simulink library "M160_lib"  (Simulink 7.8)
settings: Solver=FixedStepDiscrete  StartTime=0.0  StopTime=10.0  RelTol=1e-3
PreLoadFcn:
  | update_path
undefined symbols (not defined in the file): Afr_atCool2facLambdaReqCorr_CUR_x, Afr_atCool2facLambdaReqCorr_CUR_y, Afr_atMani2facLambdaReqCorr_CUR_x, Afr_atMani2facLambdaReqCorr_CUR_y, Afr_facLambdaReqMan, Afr_facRatioMan, Afr_facStoich, Afr_flgLambdaReqOverride, Afr_flgRatioOverride, Afr_rpmEngSpdfacRelAir2facLambdaReqBase_MAP_x, Afr_rpmEngSpdfacRelAir2facLambdaReqBase_MAP_y, Afr_rpmEngSpdfacRelAir2facLambdaReqBase_MAP_z, Ais_flgAirInjReacPumpOverride, Ais_stAirInjReacPumpMan, Amc_flgAirMassFlowOverride, Amc_uSens2AirMassFlow_CUR_x, Amc_uSens2AirMassFlow_CUR_y, Amc_uSensMaxValid, Amc_uSensMinValid, Amf_facRelAirMan, Amf_flgAirMassPerStrOverride, Amf_flgRelAirOverride, Amf_flgSwitch2AirMassFlowMeter, Amf_mAirPerStrMan, Amf_pManiEngSpd2facRelAirCorr_MAP_x, Amf_pManiEngSpd2facRelAirCorr_MAP_y, Amf_pManiEngSpd2facRelAirCorr_MAP_z, Amf_rpmEngSpd2facTempCorr_CUR_x, Amf_rpmEngSpd2facTempCorr_CUR_y, Amf_shcSpecGasConst_C, Amf_volEngDisp_C, Apv_facAirPumpRateMan, Apv_factor, Apv_flgAirPumpRateOverride, Apv_tiPeriod_C, Bvc_rVoltDivHigh, Bvc_rVoltDivLow, Bvc_uBattMax, Bvc_uBattMin, CDRV_E_OK_, Cov_facChOverVlvRateMan, Cov_factor, Cov_flgChOverVlvRateOverride, Cov_tiPeriod_C, Cpc_atManiTmp2facPresCorr_CUR_x, Cpc_atManiTmp2facPresCorr_CUR_y, Cpc_flgPChargeOverride, Cpc_uSens2pManiBase_CUR_x, Cpc_uSens2pManiBase_CUR_y, Ctc_rPullUp_C, Ctc_rSens2atCool_CUR_x, Ctc_rSens2atCool_CUR_y, Ctc_uSensMaxValid, Ctc_uSensMinValid, Ctc_uSupply, Doh_OutputDiagnosisOverride, dummy_facAirPumpRateReq, dummy_facChOverVlvRateReq, dummy_flgInterCoolerOverride, dummy_flgKl50Override ... (+243)
libraries: simulink x36, ehooks_lib x3
(part 4 of 8)

== system M160_lib/Sensors/Ctc ==
  function : TriggerPort  TriggerType=function-call
  Constant : Constant  Value=Ctc_rPullUp_C
  Constant3 : Constant  Value=Ctc_uSupply
  Constant6 : Constant  Value=0  OutDataTypeStr=single
  Ctc_rSens2atCool_CUR : Lookup_n-D  NumberOfTableDimensions=1  BreakpointsForDimension1=Ctc_rSens2atCool_CUR_x  BreakpointsForDimension1DataTypeStr=Inherit: Inherit from 'Breakpoint data'  Table=Ctc_rSens2atCool_CUR_y  TableDataTypeStr=Inherit: Inherit from 'Table data'  ExtrapMethod=Clip  OutDataTypeStr=Inherit: Inherit from 'Table data'  InputSameDT=on
  Divide : Product  Inputs=*/  OutDataTypeStr=Inherit: Same as first input
  G1_ADC_Input_Receive : Subsystem  LoadFcn=ehooks_medc17flex_devlib_io_block('load');  InitFcn=ehooks_medc17flex_devlib_io_block('init');  StartFcn=ehooks_medc17flex_devlib_io_block('start');  StopFcn=ehooks_medc17flex_devlib_io_block('stop');  ClipboardFcn=ehooks_medc17flex_devlib_io_block('clipboard', 0); % Second argument just needed to indicate null block. See callback handler.  mask{ChannelName=I_A_AN10}
      mask prompts: ChannelName "Channel name"
      mask init:
      | ehooks_medc17flex_devlib_io_block('mask_init');
      settings: AttributesFormatString=Channel name: '%<ChannelName>'  CopyFcn=ehooks_medc17flex_devlib_io_block('copy');  DeleteFcn=ehooks_medc17flex_devlib_io_block('delete');  UndoDeleteFcn=ehooks_medc17flex_devlib_io_block('undo_delete');  ModelCloseFcn=ehooks_medc17flex_devlib_io_block('model_close');  PreSaveFcn=ehooks_medc17flex_devlib_io_block('pre_save');  PostSaveFcn=ehooks_medc17flex_devlib_io_block('post_save');  NameChangeFcn=ehooks_medc17flex_devlib_io_block('name_change');  DestroyFcn=ehooks_medc17flex_devlib_io_block('destroy', 0); % Second argument just needed to indicate null block. See callback handler.  OpenFcn=ehooks_medc17flex_devlib_io_block('open');  CloseFcn=ehooks_medc17flex_devlib_io_block('close');  ParentCloseFcn=ehooks_medc17flex_devlib_io_block('parent_close');  MoveFcn=ehooks_medc17flex_devlib_io_block('move');
      mask StyleString: popup(<empty>|I_A_AN01|I_A_AN02|I_A_AN03|I_A_AN05|I_A_AN06|I_A_AN07|I_A_AN08|I_A_AN10|I_A_AN11|I_A_AN12|I_A_AN13|I_A_AN14|I_A_AN15|I_A_AN16|I_A_AN17|I_A_AN18|I_A_AN19|I_A_AN20|I_A_AN21|I_A_AN23|I_A_AN32|I_A_AN35|I_A_AN36|I_A_AN37|I_A_AN39|I_A_AN100|I_A_AN101|I_A_AN103|I_A_AN104|I_A_AN105|I_A_AN106)
      mask Display: image(imread('Input_Analog.jpg'))
  Interval Test : simulink/Logic and Bit Operations/Interval Test  IntervalClosedRight=on  uplimit=Ctc_uSensMaxValid  IntervalClosedLeft=on  lowlimit=Ctc_uSensMinValid  OutDataTypeStr=boolean
  Logical Operator : Logic  Operator=NOT  AllPortsSameDT=off  OutDataTypeStr=boolean
  Logical Operator1 : Logic  Operator=NOT  AllPortsSameDT=off  OutDataTypeStr=boolean
  Logical Operator2 : Logic  Operator=NOT  AllPortsSameDT=off  OutDataTypeStr=boolean
  Logical Operator4 : Logic  Operator=OR  Inputs=3  AllPortsSameDT=off  OutDataTypeStr=boolean
  Product : Product  OutDataTypeStr=Inherit: Same as first input
  Relational Operator : RelationalOperator  Operator=>  OutDataTypeStr=boolean
  Subtract : Sum  Inputs=+-  OutDataTypeStr=Inherit: Same as first input
  Switch : Switch  Threshold=1
  Unit Delay : UnitDelay  SampleTime=-1
  Ctc_flgError : Outport
  Ctc_atCool : Outport  Port=2
  wires:
  Logical Operator4/1 -> Ctc_flgError/1  "Ctc_flgError"
  Logical Operator1/1 -> Logical Operator4/2
  Logical Operator/1 -> Logical Operator4/1
  Interval Test/1 -> Logical Operator1/1
  G1_ADC_Input_Receive/2(uRaw) -> Subtract/2, Product/1, Interval Test/1  "Ctc_uSens"
  G1_ADC_Input_Receive/1(status) -> Logical Operator/1  "Ctc_stIA"
  Constant/1 -> Product/2
  Constant3/1 -> Subtract/1
  Product/1 -> Divide/1
  Subtract/1 -> Divide/2, Relational Operator/1
  Constant6/1 -> Relational Operator/2
  Relational Operator/1 -> Logical Operator2/1, Switch/2
  Logical Operator2/1 -> Logical Operator4/3
  Switch/1 -> Ctc_atCool/1, Unit Delay/1  "Ctc_atCool"
  Unit Delay/1 -> Switch/3
  Ctc_rSens2atCool_CUR/1 -> Switch/1
  Divide/1 -> Ctc_rSens2atCool_CUR/1  "Ctc_rSens"

== system M160_lib/Sensors/Egc ==
  function : TriggerPort  TriggerType=function-call
  Abs : Abs
  Add : Sum  OutDataTypeStr=Inherit: Same as first input
  Constan1 : Constant  Value=0.05  OutDataTypeStr=single
  Constan2 : Constant  Value=0.01  OutMin=0  OutDataTypeStr=single
  Constan3 : Constant  Value=0  OutDataTypeStr=single
  Constant : Constant  Value=2  OutDataTypeStr=single
  Constant1 : Constant  Value=Egc_flgEgasOverride
  Constant2 : Constant  Value=Egc_facEgasMan
  Constant3 : Constant  Value=Egc_tiTEgasFilt
  Constant4 : Constant  Value=Egc_stEgasFilt
  Divide : Product  Inputs=*/  OutDataTypeStr=Inherit: Same as first input
  Egc_uSens2facEgas1_CUR : Lookup_n-D  NumberOfTableDimensions=1  BreakpointsForDimension1=Egc_uSens2facEgas1_CUR_x  BreakpointsForDimension1DataTypeStr=Inherit: Inherit from 'Breakpoint data'  Table=Egc_uSens2facEgas1_CUR_y  TableDataTypeStr=Inherit: Inherit from 'Table data'  ExtrapMethod=Clip  OutDataTypeStr=Inherit: Inherit from 'Table data'  InputSameDT=on
  Egc_uSens2facEgas2_CUR : Lookup_n-D  NumberOfTableDimensions=1  BreakpointsForDimension1=Egc_uSens2facEgas2_CUR_x  BreakpointsForDimension1DataTypeStr=Inherit: Inherit from 'Breakpoint data'  Table=Egc_uSens2facEgas2_CUR_y  TableDataTypeStr=Inherit: Inherit from 'Table data'  ExtrapMethod=Clip  OutDataTypeStr=Inherit: Inherit from 'Table data'  InputSameDT=on
  G1_ADC_Input_Receive : Subsystem  LoadFcn=ehooks_medc17flex_devlib_io_block('load');  InitFcn=ehooks_medc17flex_devlib_io_block('init');  StartFcn=ehooks_medc17flex_devlib_io_block('start');  StopFcn=ehooks_medc17flex_devlib_io_block('stop');  ClipboardFcn=ehooks_medc17flex_devlib_io_block('clipboard', 0); % Second argument just needed to indicate null block. See callback handler.  mask{ChannelName=I_A_AN08}
      mask prompts: ChannelName "Channel name"
      mask init:
      | ehooks_medc17flex_devlib_io_block('mask_init');
      settings: AttributesFormatString=Channel name: '%<ChannelName>'  CopyFcn=ehooks_medc17flex_devlib_io_block('copy');  DeleteFcn=ehooks_medc17flex_devlib_io_block('delete');  UndoDeleteFcn=ehooks_medc17flex_devlib_io_block('undo_delete');  ModelCloseFcn=ehooks_medc17flex_devlib_io_block('model_close');  PreSaveFcn=ehooks_medc17flex_devlib_io_block('pre_save');  PostSaveFcn=ehooks_medc17flex_devlib_io_block('post_save');  NameChangeFcn=ehooks_medc17flex_devlib_io_block('name_change');  DestroyFcn=ehooks_medc17flex_devlib_io_block('destroy', 0); % Second argument just needed to indicate null block. See callback handler.  OpenFcn=ehooks_medc17flex_devlib_io_block('open');  CloseFcn=ehooks_medc17flex_devlib_io_block('close');  ParentCloseFcn=ehooks_medc17flex_devlib_io_block('parent_close');  MoveFcn=ehooks_medc17flex_devlib_io_block('move');
      mask StyleString: popup(<empty>|I_A_AN01|I_A_AN02|I_A_AN03|I_A_AN05|I_A_AN06|I_A_AN07|I_A_AN08|I_A_AN10|I_A_AN11|I_A_AN12|I_A_AN13|I_A_AN14|I_A_AN15|I_A_AN16|I_A_AN17|I_A_AN18|I_A_AN19|I_A_AN20|I_A_AN21|I_A_AN23|I_A_AN32|I_A_AN35|I_A_AN36|I_A_AN37|I_A_AN39|I_A_AN100|I_A_AN101|I_A_AN103|I_A_AN104|I_A_AN105|I_A_AN106)
      mask Display: image(imread('Input_Analog.jpg'))
  G1_ADC_Input_Receive1 : Subsystem  LoadFcn=ehooks_medc17flex_devlib_io_block('load');  InitFcn=ehooks_medc17flex_devlib_io_block('init');  StartFcn=ehooks_medc17flex_devlib_io_block('start');  StopFcn=ehooks_medc17flex_devlib_io_block('stop');  ClipboardFcn=ehooks_medc17flex_devlib_io_block('clipboard', 0); % Second argument just needed to indicate null block. See callback handler.  mask{ChannelName=I_A_AN13}
      mask prompts: ChannelName "Channel name"
      mask init:
      | ehooks_medc17flex_devlib_io_block('mask_init');
      settings: AttributesFormatString=Channel name: '%<ChannelName>'  CopyFcn=ehooks_medc17flex_devlib_io_block('copy');  DeleteFcn=ehooks_medc17flex_devlib_io_block('delete');  UndoDeleteFcn=ehooks_medc17flex_devlib_io_block('undo_delete');  ModelCloseFcn=ehooks_medc17flex_devlib_io_block('model_close');  PreSaveFcn=ehooks_medc17flex_devlib_io_block('pre_save');  PostSaveFcn=ehooks_medc17flex_devlib_io_block('post_save');  NameChangeFcn=ehooks_medc17flex_devlib_io_block('name_change');  DestroyFcn=ehooks_medc17flex_devlib_io_block('destroy', 0); % Second argument just needed to indicate null block. See callback handler.  OpenFcn=ehooks_medc17flex_devlib_io_block('open');  CloseFcn=ehooks_medc17flex_devlib_io_block('close');  ParentCloseFcn=ehooks_medc17flex_devlib_io_block('parent_close');  MoveFcn=ehooks_medc17flex_devlib_io_block('move');
      mask StyleString: popup(<empty>|I_A_AN01|I_A_AN02|I_A_AN03|I_A_AN05|I_A_AN06|I_A_AN07|I_A_AN08|I_A_AN10|I_A_AN11|I_A_AN12|I_A_AN13|I_A_AN14|I_A_AN15|I_A_AN16|I_A_AN17|I_A_AN18|I_A_AN19|I_A_AN20|I_A_AN21|I_A_AN23|I_A_AN32|I_A_AN35|I_A_AN36|I_A_AN37|I_A_AN39|I_A_AN100|I_A_AN101|I_A_AN103|I_A_AN104|I_A_AN105|I_A_AN106)
      mask Display: image(imread('Input_Analog.jpg'))
  Interval Test : simulink/Logic and Bit Operations/Interval Test  IntervalClosedRight=on  uplimit=Egc_uSensMaxValid  IntervalClosedLeft=on  lowlimit=Egc_uSensMinValid  OutDataTypeStr=boolean
  Interval Test1 : simulink/Logic and Bit Operations/Interval Test  IntervalClosedRight=on  uplimit=Egc_uSensMaxValid  IntervalClosedLeft=on  lowlimit=Egc_uSensMinValid  OutDataTypeStr=boolean
  Logical Operator{,1..3,6} (5 alike) : Logic  Operator=NOT  AllPortsSameDT=off  OutDataTypeStr=boolean
  Logical Operator4 : Logic  Operator=OR  Inputs=5  AllPortsSameDT=off  OutDataTypeStr=boolean
  Logical Operator5 : Logic  AllPortsSameDT=off  OutDataTypeStr=boolean
  LowpassT : Subsystem
      mask Description: LowpassT
      mask Display: image(imread('LowpassT.jpg'))
  LowpassT_Fcn : Subsystem
      mask Description: LowpassT_Fcn
      mask Display: image(imread('LowpassT.jpg'))
  Manual Switch : simulink/Signal Routing/Manual Switch  sw=1  action=0  varsize=off
  Relational Oprator : RelationalOperator  Operator=>  OutDataTypeStr=boolean
  Subtract : Sum  Inputs=+-  OutDataTypeStr=Inherit: Same as first input
  Switch : Switch  Threshold=1
  Switch1 : Switch  Threshold=1
  Egc_flgError : Outport  InitialOutput=0.0
  Egc_facEgas : Outport  Port=2  InitialOutput=0.0
  wires:
  Manual Switch/1 -> Switch1/1
  LowpassT/1(Out) -> Manual Switch/1  "Egc_facEgasFilt"
  LowpassT_Fcn/1(Out) -> Manual Switch/2  "Egc_facEgasFilt_Fcn"
  Constant3/1 -> LowpassT_Fcn/3(T), LowpassT/3(T)
  Constan2/1 -> LowpassT/2(Ta)
  Constan3/1 -> LowpassT_Fcn/1(initValue), LowpassT/1(initValue)
  G1_ADC_Input_Receive1/2(uRaw) -> Egc_uSens2facEgas2_CUR/1, Interval Test1/1  "Egc_uSens2"
  G1_ADC_Input_Receive/2(uRaw) -> Egc_uSens2facEgas1_CUR/1, Interval Test/1  "Egc_uSens1"
  Divide/1 -> Switch/3  "Egc_facEgasCalc"
  G1_ADC_Input_Receive/1(status) -> Logical Operator/1  "Egc_stIA1"
  Interval Test/1 -> Logical Operator1/1
  Interval Test1/1 -> Logical Operator3/1
  Logical Operator/1 -> Logical Operator4/1
  Logical Operator1/1 -> Logical Operator4/2
  Logical Operator2/1 -> Logical Operator4/3
  Logical Operator3/1 -> Logical Operator4/4
  Logical Operator4/1 -> Logical Operator5/1
  Logical Operator5/1 -> Egc_flgError/1  "Egc_flgError"
  Egc_uSens2facEgas1_CUR/1 -> Subtract/1, Add/1  "Egc_facEgas1"
  Egc_uSens2facEgas2_CUR/1 -> Subtract/2, Add/2  "Egc_facEgas2"
  Add/1 -> Divide/1
  Constant/1 -> Divide/2
  Subtract/1 -> Abs/1
  Abs/1 -> Relational Oprator/1
  Constan1/1 -> Relational Oprator/2
  Relational Oprator/1 -> Logical Operator4/5
  Constant1/1 -> Logical Operator6/1, Switch/2
  Logical Operator6/1 -> Logical Operator5/2
  Switch/1 -> Switch1/3, LowpassT_Fcn/2(In), LowpassT/4(in)
  Switch1/1 -> Egc_facEgas/1  "Egc_facEgas"
  Constant4/1 -> Switch1/2
  G1_ADC_Input_Receive1/1(status) -> Logical Operator2/1  "Egc_stIA2"
  Constant2/1 -> Switch/1

== system M160_lib/Sensors/Klemme50 ==
  function : TriggerPort  TriggerType=function-call
  G1_Digital_Input_Receive : Subsystem  AncestorBlock=ehooks_medc17flex_G1_lib/Library Blocks/Basic_IO/Inputs/G1_Digital_Input_Receive  LoadFcn=ehooks_medc17flex_devlib_io_block('load');  InitFcn=ehooks_medc17flex_devlib_io_block('init');  StartFcn=ehooks_medc17flex_devlib_io_block('start');  StopFcn=ehooks_medc17flex_devlib_io_block('stop');  ClipboardFcn=ehooks_medc17flex_devlib_io_block('clipboard', 0); % Second argument just needed to indicate null block. See callback handler.  mask{ChannelName=I_S_DIG17}
      mask prompts: ChannelName "Channel name"
      mask init:
      | ehooks_medc17flex_devlib_io_block('mask_init');
      settings: AttributesFormatString=Channel name: '%<ChannelName>'  CopyFcn=ehooks_medc17flex_devlib_io_block('copy');  DeleteFcn=ehooks_medc17flex_devlib_io_block('delete');  UndoDeleteFcn=ehooks_medc17flex_devlib_io_block('undo_delete');  ModelCloseFcn=ehooks_medc17flex_devlib_io_block('model_close');  PreSaveFcn=ehooks_medc17flex_devlib_io_block('pre_save');  PostSaveFcn=ehooks_medc17flex_devlib_io_block('post_save');  NameChangeFcn=ehooks_medc17flex_devlib_io_block('name_change');  DestroyFcn=ehooks_medc17flex_devlib_io_block('destroy', 0); % Second argument just needed to indicate null block. See callback handler.  OpenFcn=ehooks_medc17flex_devlib_io_block('open');  CloseFcn=ehooks_medc17flex_devlib_io_block('close');  ParentCloseFcn=ehooks_medc17flex_devlib_io_block('parent_close');  MoveFcn=ehooks_medc17flex_devlib_io_block('move');
      mask StyleString: popup(<empty>|I_S_T15|I_S_DIG02|I_S_DIG05|I_S_DIG13|I_S_DIG14|I_S_DIG15|I_S_DIG16|I_S_DIG17|I_S_DIG20|I_S_DIG50)
      mask Display: image(imread('Input_Digital.jpg'))
  Logical Operator : Logic  Operator=NOT  AllPortsSameDT=off  OutDataTypeStr=boolean
  Kl50_flgError : Outport
  Kl50_stKlemme50 : Outport  Port=2
  wires:
  Logical Operator/1 -> Kl50_flgError/1  "Kl50_flgError"
  G1_Digital_Input_Receive/1(status) -> Logical Operator/1  "Kl50_stIO"
  G1_Digital_Input_Receive/2(stRaw1) -> Kl50_stKlemme50/1  "Kl50_stKlemme50"

== system M160_lib/Sensors/Mpc ==
  Epm_rpmEngSpd : Inport
  Mtc_atMani : Inport  Port=2
  Mpc_calc : Subsystem
      mask Type: Sensors
      mask Description: ManifoldPressureCalc
      mask Display:
      | image(imread('ManifoldPressure.jpg'))
      | port_label('input',1,'Epm_rpmEngSpd')
      | port_label('input',2,'Mpc_pMani')
      | port_label('input',3,'Mpc_flgError')
      | port_label('output',1,'Mpc_pManiFilt')
  Mpc_get : Subsystem
      mask Type: Sensors
      mask Description: ManifoldPressureGet
      mask Display:
      | image(imread('ManifoldPressure.jpg'))
      | port_label('input',1,'Mtc_atMani')
      | port_label('output',1,'Mpc_flgError')
      | port_label('output',2,'Mpc_pMani')
  Mpc_pMani_calc : Subsystem  Tag=ECU_FcnCallTrigger_Source  Description=|  LoadFcn=ehooks_fcncalltrigger_source_block('load');  InitFcn=ehooks_fcncalltrigger_source_block('init');  StartFcn=ehooks_fcncalltrigger_source_block('start');  StopFcn=ehooks_fcncalltrigger_source_block('stop');  ClipboardFcn=ehooks_fcncalltrigger_source_block('clipboard', 0); % Second argument just needed to indicate null block. See callback handler.  mask(ECU_FcnCallTrigger_Source){ProcessName=BypEasyhooks_S0_Pre_Proc, TaskPriority=0, TaskPeriod=1}
      | [$SL_INT_DD 20060]
      | EHOOKS ECU asynchronous function-call trigger source block.
      mask prompts: ProcessName "Process name"; TaskPriority "Task priority (0..255)"; TaskPeriod "Task sample rate (ms)"
      mask help:
      | EHOOKS ECU asynchronous function-call trigger source block.
      | The EHOOKS ECU function-call trigger source block (EHOOKS trigger block) allows Simulink model code to be integrated into the execution of the ECU software.
      mask init:
      | ehooks_fcncalltrigger_source_block('mask_init');
      settings: CopyFcn=ehooks_fcncalltrigger_source_block('copy');  DeleteFcn=ehooks_fcncalltrigger_source_block('delete');  UndoDeleteFcn=ehooks_fcncalltrigger_source_block('undo_delete');  ModelCloseFcn=ehooks_fcncalltrigger_source_block('model_close');  PreSaveFcn=ehooks_fcncalltrigger_source_block('pre_save');  PostSaveFcn=ehooks_fcncalltrigger_source_block('post_save');  NameChangeFcn=ehooks_fcncalltrigger_source_block('name_change');  DestroyFcn=ehooks_fcncalltrigger_source_block('destroy', 0); % Second argument just needed to indicate null block. See callback handler.  OpenFcn=ehooks_fcncalltrigger_source_block('open');  CloseFcn=ehooks_fcncalltrigger_source_block('close');  ParentCloseFcn=ehooks_fcncalltrigger_source_block('parent_close');  MoveFcn=ehooks_fcncalltrigger_source_block('move');
      mask Display:
      | image(imread('ehooks_fcncalltrigger_source_small.bmp', 'bmp'), [ 3 1 38 30 ])
      | port_label('Output', 1, 'BypEasyhooks_S0_Pre_Proc')
  Mpc_pMani_get : Subsystem  Tag=ECU_FcnCallTrigger_Source  Description=|  LoadFcn=ehooks_fcncalltrigger_source_block('load');  InitFcn=ehooks_fcncalltrigger_source_block('init');  StartFcn=ehooks_fcncalltrigger_source_block('start');  StopFcn=ehooks_fcncalltrigger_source_block('stop');  ClipboardFcn=ehooks_fcncalltrigger_source_block('clipboard', 0); % Second argument just needed to indicate null block. See callback handler.  mask(ECU_FcnCallTrigger_Source){ProcessName=BypEasyhooks_1ms_Pre_Proc, TaskPriority=0, TaskPeriod=1}
      | [$SL_INT_DD 20060]
      | EHOOKS ECU asynchronous function-call trigger source block.
      mask prompts: ProcessName "Process name"; TaskPriority "Task priority (0..255)"; TaskPeriod "Task sample rate (ms)"
      mask help:
      | EHOOKS ECU asynchronous function-call trigger source block.
      | The EHOOKS ECU function-call trigger source block (EHOOKS trigger block) allows Simulink model code to be integrated into the execution of the ECU software.
      mask init:
      | ehooks_fcncalltrigger_source_block('mask_init');
      settings: CopyFcn=ehooks_fcncalltrigger_source_block('copy');  DeleteFcn=ehooks_fcncalltrigger_source_block('delete');  UndoDeleteFcn=ehooks_fcncalltrigger_source_block('undo_delete');  ModelCloseFcn=ehooks_fcncalltrigger_source_block('model_close');  PreSaveFcn=ehooks_fcncalltrigger_source_block('pre_save');  PostSaveFcn=ehooks_fcncalltrigger_source_block('post_save');  NameChangeFcn=ehooks_fcncalltrigger_source_block('name_change');  DestroyFcn=ehooks_fcncalltrigger_source_block('destroy', 0); % Second argument just needed to indicate null block. See callback handler.  OpenFcn=ehooks_fcncalltrigger_source_block('open');  CloseFcn=ehooks_fcncalltrigger_source_block('close');  ParentCloseFcn=ehooks_fcncalltrigger_source_block('parent_close');  MoveFcn=ehooks_fcncalltrigger_source_block('move');
      mask Display:
      | image(imread('ehooks_fcncalltrigger_source_small.bmp', 'bmp'), [ 3 1 38 30 ])
      | port_label('Output', 1, 'BypEasyhooks_1ms_Pre_Proc')
  Mpc_flgError : Outport
  Mpc_pManiFilt : Outport  Port=2
  wires:
  Mpc_pMani_get/1(TriggerOut) -> Mpc_get/Trigger
  Mtc_atMani/1 -> Mpc_get/1(Mtc_atMani)
  Mpc_get/1(Mpc_flgError) -> Mpc_flgError/1, Mpc_calc/3(Mpc_flgError)
  Mpc_pMani_calc/1(TriggerOut) -> Mpc_calc/Trigger
  Epm_rpmEngSpd/1 -> Mpc_calc/1(Epm_rpmEngSpd)
  Mpc_get/2(Ctc_atCool1) -> Mpc_calc/2(Mpc_pMani)
  Mpc_calc/1(Mpc_pManiFilt) -> Mpc_pManiFilt/1

== system M160_lib/Sensors/Mtc ==
  function : TriggerPort  TriggerType=function-call
  Constant : Constant  Value=Mtc_rPullUp_C
  Constant3 : Constant  Value=Mtc_uSupply
  Constant6 : Constant  Value=0  OutDataTypeStr=single
  Divide : Product  Inputs=*/  OutDataTypeStr=single
  G1_ADC_Input_Receive : Subsystem  LoadFcn=ehooks_medc17flex_devlib_io_block('load');  InitFcn=ehooks_medc17flex_devlib_io_block('init');  StartFcn=ehooks_medc17flex_devlib_io_block('start');  StopFcn=ehooks_medc17flex_devlib_io_block('stop');  ClipboardFcn=ehooks_medc17flex_devlib_io_block('clipboard', 0); % Second argument just needed to indicate null block. See callback handler.  mask{ChannelName=I_A_AN14}
      mask prompts: ChannelName "Channel name"
      mask init:
      | ehooks_medc17flex_devlib_io_block('mask_init');
      settings: AttributesFormatString=Channel name: '%<ChannelName>'  CopyFcn=ehooks_medc17flex_devlib_io_block('copy');  DeleteFcn=ehooks_medc17flex_devlib_io_block('delete');  UndoDeleteFcn=ehooks_medc17flex_devlib_io_block('undo_delete');  ModelCloseFcn=ehooks_medc17flex_devlib_io_block('model_close');  PreSaveFcn=ehooks_medc17flex_devlib_io_block('pre_save');  PostSaveFcn=ehooks_medc17flex_devlib_io_block('post_save');  NameChangeFcn=ehooks_medc17flex_devlib_io_block('name_change');  DestroyFcn=ehooks_medc17flex_devlib_io_block('destroy', 0); % Second argument just needed to indicate null block. See callback handler.  OpenFcn=ehooks_medc17flex_devlib_io_block('open');  CloseFcn=ehooks_medc17flex_devlib_io_block('close');  ParentCloseFcn=ehooks_medc17flex_devlib_io_block('parent_close');  MoveFcn=ehooks_medc17flex_devlib_io_block('move');
      mask StyleString: popup(<empty>|I_A_AN01|I_A_AN02|I_A_AN03|I_A_AN05|I_A_AN06|I_A_AN07|I_A_AN08|I_A_AN10|I_A_AN11|I_A_AN12|I_A_AN13|I_A_AN14|I_A_AN15|I_A_AN16|I_A_AN17|I_A_AN18|I_A_AN19|I_A_AN20|I_A_AN21|I_A_AN23|I_A_AN32|I_A_AN35|I_A_AN36|I_A_AN37|I_A_AN39|I_A_AN100|I_A_AN101|I_A_AN103|I_A_AN104|I_A_AN105|I_A_AN106)
      mask Display: image(imread('Input_Analog.jpg'))
  Interval Test : simulink/Logic and Bit Operations/Interval Test  IntervalClosedRight=on  uplimit=Mtc_uSensMaxValid  IntervalClosedLeft=on  lowlimit=Mtc_uSensMinValid  OutDataTypeStr=boolean
  Logical Operator : Logic  Operator=NOT  AllPortsSameDT=off  OutDataTypeStr=boolean
  Logical Operator1 : Logic  Operator=NOT  AllPortsSameDT=off  OutDataTypeStr=boolean
  Logical Operator2 : Logic  Operator=NOT  AllPortsSameDT=off  OutDataTypeStr=boolean
  Logical Operator4 : Logic  Operator=OR  Inputs=3  AllPortsSameDT=off  OutDataTypeStr=boolean
  Mtc_rSens2atMani_CUR : Lookup_n-D  NumberOfTableDimensions=1  BreakpointsForDimension1=Mtc_rSens2atMani_CUR_x  BreakpointsForDimension1DataTypeStr=Inherit: Inherit from 'Breakpoint data'  Table=Mtc_rSens2atMani_CUR_y  TableDataTypeStr=Inherit: Inherit from 'Table data'  ExtrapMethod=Clip  OutDataTypeStr=Inherit: Inherit from 'Table data'  InputSameDT=on
  Product : Product  OutDataTypeStr=Inherit: Same as first input
  Relational Operator : RelationalOperator  Operator=>  OutDataTypeStr=boolean
  Subtract : Sum  Inputs=+-  OutDataTypeStr=Inherit: Same as first input
  Switch : Switch  Threshold=1
  Unit Delay : UnitDelay  SampleTime=-1
  Mtc_flgError : Outport
  Mtc_atMani : Outport  Port=2
  wires:
  Mtc_rSens2atMani_CUR/1 -> Switch/1
  Unit Delay/1 -> Switch/3
  Switch/1 -> Unit Delay/1, Mtc_atMani/1  "Mtc_atMani"
  Logical Operator2/1 -> Logical Operator4/3
  Divide/1 -> Mtc_rSens2atMani_CUR/1  "Mtc_rSens"
  Relational Operator/1 -> Switch/2, Logical Operator2/1
  Constant6/1 -> Relational Operator/2
  Subtract/1 -> Relational Operator/1, Divide/2
  Product/1 -> Divide/1
  Constant3/1 -> Subtract/1
  Constant/1 -> Product/2
  G1_ADC_Input_Receive/1(status) -> Logical Operator/1  "Mtc_stIA"
  G1_ADC_Input_Receive/2(uRaw) -> Product/1, Subtract/2, Interval Test/1  "Mtc_uSens"
  Interval Test/1 -> Logical Operator1/1
  Logical Operator/1 -> Logical Operator4/1
  Logical Operator1/1 -> Logical Operator4/2
  Logical Operator4/1 -> Mtc_flgError/1  "Mtc_flgError"

== system M160_lib/Sensors/Opc ==
  Epm_rpmEngSpd : Inport
  function : TriggerPort  TriggerType=function-call
  Constant : Constant  Value=Opc_rpmEngMinOilPressure
  G1_Digital_Input_Receive : Subsystem  AncestorBlock=ehooks_medc17flex_G1_lib/Library Blocks/Basic_IO/Inputs/G1_Digital_Input_Receive  LoadFcn=ehooks_medc17flex_devlib_io_block('load');  InitFcn=ehooks_medc17flex_devlib_io_block('init');  StartFcn=ehooks_medc17flex_devlib_io_block('start');  StopFcn=ehooks_medc17flex_devlib_io_block('stop');  ClipboardFcn=ehooks_medc17flex_devlib_io_block('clipboard', 0); % Second argument just needed to indicate null block. See callback handler.  mask{ChannelName=I_S_DIG13}
      mask prompts: ChannelName "Channel name"
      mask init:
      | ehooks_medc17flex_devlib_io_block('mask_init');
      settings: AttributesFormatString=Channel name: '%<ChannelName>'  CopyFcn=ehooks_medc17flex_devlib_io_block('copy');  DeleteFcn=ehooks_medc17flex_devlib_io_block('delete');  UndoDeleteFcn=ehooks_medc17flex_devlib_io_block('undo_delete');  ModelCloseFcn=ehooks_medc17flex_devlib_io_block('model_close');  PreSaveFcn=ehooks_medc17flex_devlib_io_block('pre_save');  PostSaveFcn=ehooks_medc17flex_devlib_io_block('post_save');  NameChangeFcn=ehooks_medc17flex_devlib_io_block('name_change');  DestroyFcn=ehooks_medc17flex_devlib_io_block('destroy', 0); % Second argument just needed to indicate null block. See callback handler.  OpenFcn=ehooks_medc17flex_devlib_io_block('open');  CloseFcn=ehooks_medc17flex_devlib_io_block('close');  ParentCloseFcn=ehooks_medc17flex_devlib_io_block('parent_close');  MoveFcn=ehooks_medc17flex_devlib_io_block('move');
      mask StyleString: popup(<empty>|I_S_T15|I_S_DIG02|I_S_DIG05|I_S_DIG13|I_S_DIG14|I_S_DIG15|I_S_DIG16|I_S_DIG17|I_S_DIG20|I_S_DIG50)
      mask Display: image(imread('Input_Digital.jpg'))
  Gain : Gain  OutDataTypeStr=Inherit: Same as input
  Logical Operator : Logic  Operator=NOT  AllPortsSameDT=off  OutDataTypeStr=boolean
  Logical Operator1 : Logic  Operator=NOT  AllPortsSameDT=off  OutDataTypeStr=boolean
  Logical Operator3 : Logic  AllPortsSameDT=off  OutDataTypeStr=boolean
  Logical Operator4 : Logic  Operator=OR  AllPortsSameDT=off  OutDataTypeStr=boolean
  Relational Operator : RelationalOperator  Operator=>  OutDataTypeStr=boolean
  Opc_flgError : Outport
  Opc_stOilPressure : Outport  Port=2
  wires:
  Gain/1 -> Opc_stOilPressure/1  "Opc_stOilPressure"
  Constant/1 -> Relational Operator/2
  Logical Operator4/1 -> Opc_flgError/1  "Opc_flgError"
  Logical Operator/1 -> Logical Operator4/1
  G1_Digital_Input_Receive/1(status) -> Logical Operator/1  "Opc_stIA"
  Epm_rpmEngSpd/1 -> Relational Operator/1
  Relational Operator/1 -> Logical Operator3/1
  Logical Operator3/1 -> Logical Operator4/2
  Logical Operator1/1 -> Logical Operator3/2
  G1_Digital_Input_Receive/2(stRaw1) -> Logical Operator1/1, Gain/1  "Opc_stSens"

== system M160_lib/Actuators/Ais/G1_DigOut_Ctrl ==
  state : Inport
  DTC_DigOut_ctrl : DataTypeConversion  OutDataTypeStr=uint8  RndMeth=Nearest
  DTC_Out1 : DataTypeConversion  OutDataTypeStr=boolean
  FlexECU_DevLib_FcnAPI_Wrapper_SFcn : S-Function  FunctionName=ehooks_medc17flex_devlib_basic_io_fcncall  Parameters=NoInputPorts, NoOutputPorts, InputPortDataTypes, OutputPortDataTypes, CFunctionArgTypes, CFunctionName, ChannelName  EnableBusSupport=off  mask{NoInputPorts=1, NoOutputPorts=1, InputPortDataTypes=uint8, OutputPortDataTypes=uint8, CFunctionArgTypes=ret,val, CFunctionName=DevLib_Dio_Set, ChannelName=O_S_RL30}
      mask prompts: NoInputPorts "Number of input ports"; NoOutputPorts "Number of output ports"; InputPortDataTypes "Input port data types"; OutputPortDataTypes "Output port data types"; CFunctionArgTypes "C function argument types"; CFunctionName "C function name"; ChannelName "Channel (pin) name"
      mask Display: disp('EHOOKS FlexECU\nDevLib Wrapper\nS-Function')
  status : Outport
  wires:
  DTC_Out1/1 -> status/1
  FlexECU_DevLib_FcnAPI_Wrapper_SFcn/1 -> DTC_Out1/1
  state/1 -> DTC_DigOut_ctrl/1
  DTC_DigOut_ctrl/1 -> FlexECU_DevLib_FcnAPI_Wrapper_SFcn/1

== system M160_lib/Actuators/Ais/G1_DigOut_GetError ==
  DTC_DigOut_GetError : DataTypeConversion  OutDataTypeStr=single
  FlexECU_DevLib_FcnAPI_Wrapper_SFcn : S-Function  FunctionName=ehooks_medc17flex_devlib_basic_io_fcncall  Parameters=NoInputPorts, NoOutputPorts, InputPortDataTypes, OutputPortDataTypes, CFunctionArgTypes, CFunctionName, ChannelName  EnableBusSupport=off  mask{NoInputPorts=0, NoOutputPorts=1, InputPortDataTypes=, OutputPortDataTypes=uint8, CFunctionArgTypes=ret, CFunctionName=DevLib_DioSet_GetError, ChannelName=O_S_RL30}
      mask prompts: NoInputPorts "Number of input ports"; NoOutputPorts "Number of output ports"; InputPortDataTypes "Input port data types"; OutputPortDataTypes "Output port data types"; CFunctionArgTypes "C function argument types"; CFunctionName "C function name"; ChannelName "Channel (pin) name"
      mask Display: disp('EHOOKS FlexECU\nDevLib Wrapper\nS-Function')
  status : Outport
  wires:
  FlexECU_DevLib_FcnAPI_Wrapper_SFcn/1 -> DTC_DigOut_GetError/1
  DTC_DigOut_GetError/1 -> status/1

== system M160_lib/Actuators/Apv/G1_PWM_Output_Ctrl ==
  dutycycle : Inport
  period : Inport  Port=2
  factor : Inport  Port=3
  level : Inport  Port=4
  DTC_PwmOut_DutyCycle : DataTypeConversion  OutDataTypeStr=int16  RndMeth=Nearest
  DTC_PwmOut_ErrorInfo : DataTypeConversion  OutDataTypeStr=boolean
  DTC_PwmOut_Level : DataTypeConversion  OutDataTypeStr=int16  RndMeth=Nearest
  DTC_PwmOut_Period : DataTypeConversion  OutDataTypeStr=int16  RndMeth=Nearest
  DTC_PwmOut_Period1 : DataTypeConversion  OutDataTypeStr=uint8  RndMeth=Nearest
  FlexECU_DevLib_FcnAPI_Wrapper_SFcn : S-Function  FunctionName=ehooks_medc17flex_devlib_basic_io_fcncall  Parameters=NoInputPorts, NoOutputPorts, InputPortDataTypes, OutputPortDataTypes, CFunctionArgTypes, CFunctionName, ChannelName  EnableBusSupport=off  mask{NoInputPorts=4, NoOutputPorts=1, InputPortDataTypes=int16,int16, int16, uint8, OutputPortDataTypes=uint8, CFunctionArgTypes=ret,val,val,val,val, CFunctionName=DevLib_Pwm_Out, ChannelName=O_T_RL13}
      mask prompts: NoInputPorts "Number of input ports"; NoOutputPorts "Number of output ports"; InputPortDataTypes "Input port data types"; OutputPortDataTypes "Output port data types"; CFunctionArgTypes "C function argument types"; CFunctionName "C function name"; ChannelName "Channel (pin) name"
      mask Display: disp('EHOOKS FlexECU\nDevLib Wrapper\nS-Function')
  Gain : Gain  Gain=100
  status : Outport
  wires:
  DTC_PwmOut_ErrorInfo/1 -> status/1
  DTC_PwmOut_Level/1 -> FlexECU_DevLib_FcnAPI_Wrapper_SFcn/3
  DTC_PwmOut_Period/1 -> FlexECU_DevLib_FcnAPI_Wrapper_SFcn/2
  DTC_PwmOut_DutyCycle/1 -> FlexECU_DevLib_FcnAPI_Wrapper_SFcn/1
  factor/1 -> DTC_PwmOut_Level/1
  period/1 -> DTC_PwmOut_Period/1
  FlexECU_DevLib_FcnAPI_Wrapper_SFcn/1 -> DTC_PwmOut_ErrorInfo/1
  DTC_PwmOut_Period1/1 -> FlexECU_DevLib_FcnAPI_Wrapper_SFcn/4
  level/1 -> DTC_PwmOut_Period1/1
  dutycycle/1 -> Gain/1
  Gain/1 -> DTC_PwmOut_DutyCycle/1

== system M160_lib/Actuators/Apv/G1_PwmOut_Get_error ==
  DTC_PwmOut_GetError : DataTypeConversion  OutDataTypeStr=single
  FlexECU_DevLib_FcnAPI_Wrapper_SFcn : S-Function  FunctionName=ehooks_medc17flex_devlib_basic_io_fcncall  Parameters=NoInputPorts, NoOutputPorts, InputPortDataTypes, OutputPortDataTypes, CFunctionArgTypes, CFunctionName, ChannelName  EnableBusSupport=off  mask{NoInputPorts=0, NoOutputPorts=1, InputPortDataTypes=, OutputPortDataTypes=uint8, CFunctionArgTypes=ret, CFunctionName=DevLib_PwmOut_GetError, ChannelName=O_T_RL13}
      mask prompts: NoInputPorts "Number of input ports"; NoOutputPorts "Number of output ports"; InputPortDataTypes "Input port data types"; OutputPortDataTypes "Output port data types"; CFunctionArgTypes "C function argument types"; CFunctionName "C function name"; ChannelName "Channel (pin) name"
      mask Display: disp('EHOOKS FlexECU\nDevLib Wrapper\nS-Function')
  status : Outport
  wires:
  FlexECU_DevLib_FcnAPI_Wrapper_SFcn/1 -> DTC_PwmOut_GetError/1
  DTC_PwmOut_GetError/1 -> status/1

== system M160_lib/Actuators/Cov/G1_PWM_Output_Ctrl ==
  dutycycle : Inport
  period : Inport  Port=2
  factor : Inport  Port=3
  level : Inport  Port=4
  DTC_PwmOut_DutyCycle : DataTypeConversion  OutDataTypeStr=int16  RndMeth=Nearest
  DTC_PwmOut_ErrorInfo : DataTypeConversion  OutDataTypeStr=boolean
  DTC_PwmOut_Level : DataTypeConversion  OutDataTypeStr=int16  RndMeth=Nearest
  DTC_PwmOut_Period : DataTypeConversion  OutDataTypeStr=int16  RndMeth=Nearest
  DTC_PwmOut_Period1 : DataTypeConversion  OutDataTypeStr=uint8  RndMeth=Nearest
  FlexECU_DevLib_FcnAPI_Wrapper_SFcn : S-Function  FunctionName=ehooks_medc17flex_devlib_basic_io_fcncall  Parameters=NoInputPorts, NoOutputPorts, InputPortDataTypes, OutputPortDataTypes, CFunctionArgTypes, CFunctionName, ChannelName  EnableBusSupport=off  mask{NoInputPorts=4, NoOutputPorts=1, InputPortDataTypes=int16,int16, int16, uint8, OutputPortDataTypes=uint8, CFunctionArgTypes=ret,val,val,val,val, CFunctionName=DevLib_Pwm_Out, ChannelName=O_T_RL10}
      mask prompts: NoInputPorts "Number of input ports"; NoOutputPorts "Number of output ports"; InputPortDataTypes "Input port data types"; OutputPortDataTypes "Output port data types"; CFunctionArgTypes "C function argument types"; CFunctionName "C function name"; ChannelName "Channel (pin) name"
      mask Display: disp('EHOOKS FlexECU\nDevLib Wrapper\nS-Function')
  Gain : Gain  Gain=100
  status : Outport
  wires:
  Gain/1 -> DTC_PwmOut_DutyCycle/1
  dutycycle/1 -> Gain/1
  level/1 -> DTC_PwmOut_Period1/1
  DTC_PwmOut_Period1/1 -> FlexECU_DevLib_FcnAPI_Wrapper_SFcn/4
  FlexECU_DevLib_FcnAPI_Wrapper_SFcn/1 -> DTC_PwmOut_ErrorInfo/1
  period/1 -> DTC_PwmOut_Period/1
  factor/1 -> DTC_PwmOut_Level/1
  DTC_PwmOut_DutyCycle/1 -> FlexECU_DevLib_FcnAPI_Wrapper_SFcn/1
  DTC_PwmOut_Period/1 -> FlexECU_DevLib_FcnAPI_Wrapper_SFcn/2
  DTC_PwmOut_Level/1 -> FlexECU_DevLib_FcnAPI_Wrapper_SFcn/3
  DTC_PwmOut_ErrorInfo/1 -> status/1

== system M160_lib/Actuators/Cov/G1_PwmOut_Get_error ==
  DTC_PwmOut_GetError : DataTypeConversion  OutDataTypeStr=single
  FlexECU_DevLib_FcnAPI_Wrapper_SFcn : S-Function  FunctionName=ehooks_medc17flex_devlib_basic_io_fcncall  Parameters=NoInputPorts, NoOutputPorts, InputPortDataTypes, OutputPortDataTypes, CFunctionArgTypes, CFunctionName, ChannelName  EnableBusSupport=off  mask{NoInputPorts=0, NoOutputPorts=1, InputPortDataTypes=, OutputPortDataTypes=uint8, CFunctionArgTypes=ret, CFunctionName=DevLib_PwmOut_GetError, ChannelName=O_T_RL10}
      mask prompts: NoInputPorts "Number of input ports"; NoOutputPorts "Number of output ports"; InputPortDataTypes "Input port data types"; OutputPortDataTypes "Output port data types"; CFunctionArgTypes "C function argument types"; CFunctionName "C function name"; ChannelName "Channel (pin) name"
      mask Display: disp('EHOOKS FlexECU\nDevLib Wrapper\nS-Function')
  status : Outport
  wires:
  DTC_PwmOut_GetError/1 -> status/1
  FlexECU_DevLib_FcnAPI_Wrapper_SFcn/1 -> DTC_PwmOut_GetError/1

== system M160_lib/Actuators/Fps/G1_DigOut_Ctrl ==
  state : Inport
  DTC_DigOut_ctrl : DataTypeConversion  OutDataTypeStr=uint8  RndMeth=Nearest
  DTC_Out1 : DataTypeConversion  OutDataTypeStr=boolean
  FlexECU_DevLib_FcnAPI_Wrapper_SFcn : S-Function  FunctionName=ehooks_medc17flex_devlib_basic_io_fcncall  Parameters=NoInputPorts, NoOutputPorts, InputPortDataTypes, OutputPortDataTypes, CFunctionArgTypes, CFunctionName, ChannelName  EnableBusSupport=off  mask{NoInputPorts=1, NoOutputPorts=1, InputPortDataTypes=uint8, OutputPortDataTypes=uint8, CFunctionArgTypes=ret,val, CFunctionName=DevLib_Dio_Set, ChannelName=O_S_RL09}
      mask prompts: NoInputPorts "Number of input ports"; NoOutputPorts "Number of output ports"; InputPortDataTypes "Input port data types"; OutputPortDataTypes "Output port data types"; CFunctionArgTypes "C function argument types"; CFunctionName "C function name"; ChannelName "Channel (pin) name"
      mask Display: disp('EHOOKS FlexECU\nDevLib Wrapper\nS-Function')
  status : Outport
  wires:
  DTC_Out1/1 -> status/1
  FlexECU_DevLib_FcnAPI_Wrapper_SFcn/1 -> DTC_Out1/1
  state/1 -> DTC_DigOut_ctrl/1
  DTC_DigOut_ctrl/1 -> FlexECU_DevLib_FcnAPI_Wrapper_SFcn/1

== system M160_lib/Actuators/Fps/G1_DigOut_GetError ==
  DTC_DigOut_GetError : DataTypeConversion  OutDataTypeStr=single
  FlexECU_DevLib_FcnAPI_Wrapper_SFcn : S-Function  FunctionName=ehooks_medc17flex_devlib_basic_io_fcncall  Parameters=NoInputPorts, NoOutputPorts, InputPortDataTypes, OutputPortDataTypes, CFunctionArgTypes, CFunctionName, ChannelName  EnableBusSupport=off  mask{NoInputPorts=0, NoOutputPorts=1, InputPortDataTypes=, OutputPortDataTypes=uint8, CFunctionArgTypes=ret, CFunctionName=DevLib_DioSet_GetError, ChannelName=O_S_RL09}
      mask prompts: NoInputPorts "Number of input ports"; NoOutputPorts "Number of output ports"; InputPortDataTypes "Input port data types"; OutputPortDataTypes "Output port data types"; CFunctionArgTypes "C function argument types"; CFunctionName "C function name"; ChannelName "Channel (pin) name"
      mask Display: disp('EHOOKS FlexECU\nDevLib Wrapper\nS-Function')
  status : Outport
  wires:
  FlexECU_DevLib_FcnAPI_Wrapper_SFcn/1 -> DTC_DigOut_GetError/1
  DTC_DigOut_GetError/1 -> status/1

== system M160_lib/Actuators/Icc/EdgeFalling ==
  signal : Inport
  Detect Decrease : simulink/Logic and Bit Operations/Detect Decrease  vinit=0.0  InputProcessing=Inherited  OutDataTypeStr=boolean
  return : Outport
  wires:
  signal/1 -> Detect Decrease/1
  Detect Decrease/1 -> return/1

== system M160_lib/Actuators/Icc/EdgeRising ==
  signal : Inport
  Detect Increase : simulink/Logic and Bit Operations/Detect Increase  vinit=0.0  InputProcessing=Inherited  OutDataTypeStr=boolean
  return : Outport
  wires:
  signal/1 -> Detect Increase/1
  Detect Increase/1 -> return/1

== system M160_lib/Actuators/Icc/G1_IGN_SetParam_for_PFI ==
  szout_w : Inport
  szfuba_w : Inport  Port=2
  offz_w : Inport  Port=3
  IGN_zwcalcar_1 : Inport  Port=4
  IGN_zwcalcar_2 : Inport  Port=5
  IGN_zwcalcar_3 : Inport  Port=6
  IGN_zwcalcar_4 : Inport  Port=7
  IGN_zwcalcar_5 : Inport  Port=8
  IGN_zwcalcar_6 : Inport  Port=9
  IGN_zwcalcar_7 : Inport  Port=10
  IGN_zwcalcar_8 : Inport  Port=11
  IGN_fubaanz : Inport  Port=12
  DTC_IGN_fubaanz : DataTypeConversion  OutDataTypeStr=uint8  RndMeth=Nearest
  DTC_IGN_offz_w : DataTypeConversion  OutDataTypeStr=uint16  RndMeth=Nearest
  DTC_IGN_szfuba_w : DataTypeConversion  OutDataTypeStr=uint16  RndMeth=Nearest
  DTC_IGN_szout_w : DataTypeConversion  OutDataTypeStr=uint16  RndMeth=Nearest
  DTC_IGN_zwcalcar4 : DataTypeConversion  OutDataTypeStr=int8  RndMeth=Nearest
  DTC_IGN_zwcalcar_{1..3,5..8} (7 alike) : DataTypeConversion  OutDataTypeStr=int8  RndMeth=Nearest
  DTC_PFI_CdrvError : DataTypeConversion  OutDataTypeStr=single
  FlexECU_SFcn_PFI_Ign : S-Function  FunctionName=ehooks_medc17flex_devlib_ign_struct_fcncall  Parameters=NoInputPorts, NoOutputPorts, InputPortDataTypes, OutputPortDataTypes, CFunctionArgTypes, CFunctionName, StructMemberNames, StructTypeName, InputPortDataWidths, OutputPortDataWidths  EnableBusSupport=off  mask{NoInputPorts=5, NoOutputPorts=1, InputPortDataTypes=uint16, uint16, uint16, int8,uint8, OutputPortDataTypes=uint8, CFunctionArgTypes=ret,val, val, val, refin, val, CFunctionName=IgnCl_PfiSetParam, StructMemberNames=szout_w, szfuba_w, offz_w, zwcalcar, fubaanz, StructTypeName=IgnClInterface_type, InputPortDataWidths=1,1,1,8,1, OutputPortDataWidths=1}
      mask prompts: NoInputPorts "Number of input ports"; NoOutputPorts "Number of output ports"; InputPortDataTypes "Input port data types"; OutputPortDataTypes "Output port data types"; CFunctionArgTypes "C function argument types"; CFunctionName "C function name"; StructMemberNames "Structure member names"; StructTypeName "Structure type name"; InputPortDataWidths "Input port widths"; OutputPortDataWidths "Output port widths"
      mask Display: disp('EHOOKS FlexECU\nDevLib Wrapper\nS-Function')
  Mux : Mux  Inputs=8
  status : Outport
  wires:
  DTC_PFI_CdrvError/1 -> status/1
  FlexECU_SFcn_PFI_Ign/1 -> DTC_PFI_CdrvError/1
  DTC_IGN_offz_w/1 -> FlexECU_SFcn_PFI_Ign/3
  szout_w/1 -> DTC_IGN_szout_w/1
  DTC_IGN_zwcalcar_1/1 -> Mux/1
  Mux/1 -> FlexECU_SFcn_PFI_Ign/4  "tez_xxx"
  szfuba_w/1 -> DTC_IGN_szfuba_w/1
  DTC_IGN_szfuba_w/1 -> FlexECU_SFcn_PFI_Ign/2
  offz_w/1 -> DTC_IGN_offz_w/1
  IGN_zwcalcar_1/1 -> DTC_IGN_zwcalcar_1/1
  DTC_IGN_fubaanz/1 -> FlexECU_SFcn_PFI_Ign/5
  DTC_IGN_zwcalcar_2/1 -> Mux/2
  IGN_zwcalcar_2/1 -> DTC_IGN_zwcalcar_2/1
  DTC_IGN_zwcalcar_3/1 -> Mux/3
  IGN_zwcalcar_3/1 -> DTC_IGN_zwcalcar_3/1
  DTC_IGN_zwcalcar4/1 -> Mux/4
  IGN_zwcalcar_4/1 -> DTC_IGN_zwcalcar4/1
  DTC_IGN_zwcalcar_5/1 -> Mux/5
  IGN_zwcalcar_5/1 -> DTC_IGN_zwcalcar_5/1
  DTC_IGN_zwcalcar_6/1 -> Mux/6
  IGN_zwcalcar_6/1 -> DTC_IGN_zwcalcar_6/1
  DTC_IGN_zwcalcar_7/1 -> Mux/7
  IGN_zwcalcar_7/1 -> DTC_IGN_zwcalcar_7/1
  DTC_IGN_zwcalcar_8/1 -> Mux/8
  IGN_zwcalcar_8/1 -> DTC_IGN_zwcalcar_8/1
  IGN_fubaanz/1 -> DTC_IGN_fubaanz/1
  DTC_IGN_szout_w/1 -> FlexECU_SFcn_PFI_Ign/1

== system M160_lib/Actuators/Icc/IGN_FadeOut_Immediate ==
  FlexECU_SFcn_Frm_CAN_Init : S-Function  Priority=48  FunctionName=ehooks_medc17flex_devlib_CAN_Init_fcncall  Parameters=CFunctionName  EnableBusSupport=off  mask{CFunctionName=IgnCl_fadeOutImmediate}
      mask prompts: CFunctionName "C function name"
      mask Display: disp('EHOOKS FlexECU\nDevLib Wrapper\nS-Function')

== system M160_lib/Actuators/Ics/G1_DigOut_Ctrl ==
  state : Inport
  DTC_DigOut_ctrl : DataTypeConversion  OutDataTypeStr=uint8  RndMeth=Nearest
  DTC_Out1 : DataTypeConversion  OutDataTypeStr=boolean
  FlexECU_DevLib_FcnAPI_Wrapper_SFcn : S-Function  FunctionName=ehooks_medc17flex_devlib_basic_io_fcncall  Parameters=NoInputPorts, NoOutputPorts, InputPortDataTypes, OutputPortDataTypes, CFunctionArgTypes, CFunctionName, ChannelName  EnableBusSupport=off  mask{NoInputPorts=1, NoOutputPorts=1, InputPortDataTypes=uint8, OutputPortDataTypes=uint8, CFunctionArgTypes=ret,val, CFunctionName=DevLib_Dio_Set, ChannelName=O_S_RL29}
      mask prompts: NoInputPorts "Number of input ports"; NoOutputPorts "Number of output ports"; InputPortDataTypes "Input port data types"; OutputPortDataTypes "Output port data types"; CFunctionArgTypes "C function argument types"; CFunctionName "C function name"; ChannelName "Channel (pin) name"
      mask Display: disp('EHOOKS FlexECU\nDevLib Wrapper\nS-Function')
  status : Outport
  wires:
  DTC_DigOut_ctrl/1 -> FlexECU_DevLib_FcnAPI_Wrapper_SFcn/1
  state/1 -> DTC_DigOut_ctrl/1
  FlexECU_DevLib_FcnAPI_Wrapper_SFcn/1 -> DTC_Out1/1
  DTC_Out1/1 -> status/1

== system M160_lib/Actuators/Ics/G1_DigOut_GetError ==
  DTC_DigOut_GetError : DataTypeConversion  OutDataTypeStr=single
  FlexECU_DevLib_FcnAPI_Wrapper_SFcn : S-Function  FunctionName=ehooks_medc17flex_devlib_basic_io_fcncall  Parameters=NoInputPorts, NoOutputPorts, InputPortDataTypes, OutputPortDataTypes, CFunctionArgTypes, CFunctionName, ChannelName  EnableBusSupport=off  mask{NoInputPorts=0, NoOutputPorts=1, InputPortDataTypes=, OutputPortDataTypes=uint8, CFunctionArgTypes=ret, CFunctionName=DevLib_DioSet_GetError, ChannelName=O_S_RL29}
      mask prompts: NoInputPorts "Number of input ports"; NoOutputPorts "Number of output ports"; InputPortDataTypes "Input port data types"; OutputPortDataTypes "Output port data types"; CFunctionArgTypes "C function argument types"; CFunctionName "C function name"; ChannelName "Channel (pin) name"
      mask Display: disp('EHOOKS FlexECU\nDevLib Wrapper\nS-Function')
  status : Outport
  wires:
  DTC_DigOut_GetError/1 -> status/1
  FlexECU_DevLib_FcnAPI_Wrapper_SFcn/1 -> DTC_DigOut_GetError/1
